simulink model "Q2block"  (R2020b)
settings: Solver=VariableStepAuto  StartTime=0.0  StopTime=10.0  RelTol=1e-3
libraries: cstblocks x4
settings Model: Creator=HASEE  LastModifiedBy=47845

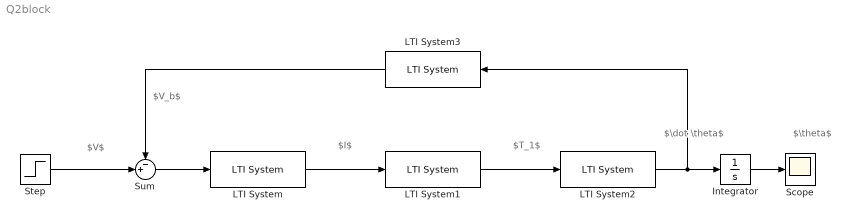
== system Q2block ==
  note: $V$
  note: $V_b$
  note: $I$
  note: $\dot \theta$
  note: $T_1$
  note: $\theta$
  Integrator : Integrator
  LTI System : cstblocks/LTI System  sys=G3  IC=[]
  LTI System1 : cstblocks/LTI System  sys=G4  IC=[]
  LTI System2 : cstblocks/LTI System  sys=G5  IC=[]
  LTI System3 : cstblocks/LTI System  sys=G6  IC=[]
  Scope : Scope
  Step : Step  SampleTime=0
  Sum : Sum  Inputs=-+|
  wires:
  LTI System/1 -> LTI System1/1
  LTI System1/1 -> LTI System2/1
  LTI System2/1 -> Integrator/1, LTI System3/1
  Sum/1 -> LTI System/1
  LTI System3/1 -> Sum/1
  Integrator/1 -> Scope/1
  Step/1 -> Sum/2
